simulink model "rockoon_2D_Launch"  (R2013a)
settings: Solver=ode45  StartTime=0.0  StopTime=t_end  RelTol=1e-3
values from neighbouring files (symbols this model uses):
  sx_0 = 0    [rockoon_launch.m]
  sy_0 = 70000 * 0.3048    (= 21336)    [rockoon_launch.m]
  theta_0 = 90    [rockoon_launch.m]
  theta_dot_0 = 20    [rockoon_launch.m]
  vx_0 = 0    [rockoon_launch.m]
  vy_0 = 0.0000001    (= 1e-07)    [rockoon_launch.m]
settings Model: Creator=Willdog  LastModifiedBy=Willdog

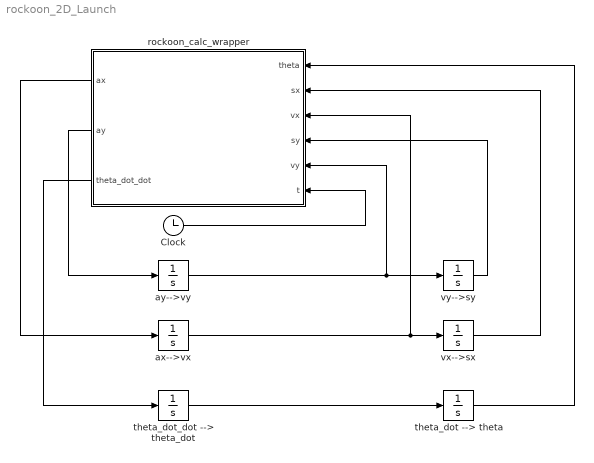
== system rockoon_2D_Launch ==
  Clock : Clock
  ax-->vx : Integrator  InitialCondition=vx_0
  ay-->vy : Integrator  InitialCondition=vy_0
  rockoon_calc_wrapper : MATLAB Function  TreatAsAtomicUnit=on
  theta_dot --> theta : Integrator  InitialCondition=theta_0
  theta_dot_dot --> theta_dot : Integrator  InitialCondition=theta_dot_0
  vx-->sx : Integrator  InitialCondition=sx_0
  vy-->sy : Integrator  InitialCondition=sy_0
  wires:
  ax-->vx/1 -> rockoon_calc_wrapper/3(vx), vx-->sx/1
  theta_dot_dot --> theta_dot/1 -> theta_dot --> theta/1
  theta_dot --> theta/1 -> rockoon_calc_wrapper/1(theta)
  vx-->sx/1 -> rockoon_calc_wrapper/2(sx)
  rockoon_calc_wrapper/3(theta_dot_dot) -> theta_dot_dot --> theta_dot/1
  rockoon_calc_wrapper/1(ax) -> ax-->vx/1
  rockoon_calc_wrapper/2(ay) -> ay-->vy/1
  ay-->vy/1 -> rockoon_calc_wrapper/5(vy), vy-->sy/1
  vy-->sy/1 -> rockoon_calc_wrapper/4(sy)
  Clock/1 -> rockoon_calc_wrapper/6(t)

== matlab function rockoon_2D_Launch/rockoon_calc_wrapper ==
  data: theta input; ax output; ay output; sx input; vx input; theta_dot_dot output; sy input; vy input; t input
function [ax,ay,theta_dot_dot] = rockoon_calc_wrapper(theta,sx,vx,sy,vy,t)

%declare extrinsic function and sync global variables
coder.extrinsic('-sync:on', 'rockoon_calc');

%init variable space
ax = 0;
ay = 0;
theta_dot_dot = 0;

%call function in matlab
[ax,ay,theta_dot_dot] = rockoon_calc(theta,sx,vx,sy,vy,t);


end
